simulink model "rosplotlive2018a"  (R2018a)
settings: Solver=VariableStepAuto  StartTime=0.0  StopTime=inf  RelTol=1e-3
undefined symbols (not defined in the file or in its folder): KDalt, KDphi, KDtheta, KIalt, KIp, KIphi, KIq, KIr, KItheta, KNalt, KPalt, KPp, KPphi, KPq, KPr, KPtheta
libraries: robotlib x8, aerolibanimutils x1
settings Model: Creator=Luca  LastModifiedBy=Arne
settings DebuggingCC: LibraryContextMissingDiagnostic=warning
settings CodeAppCC: StateflowObjectComments=on

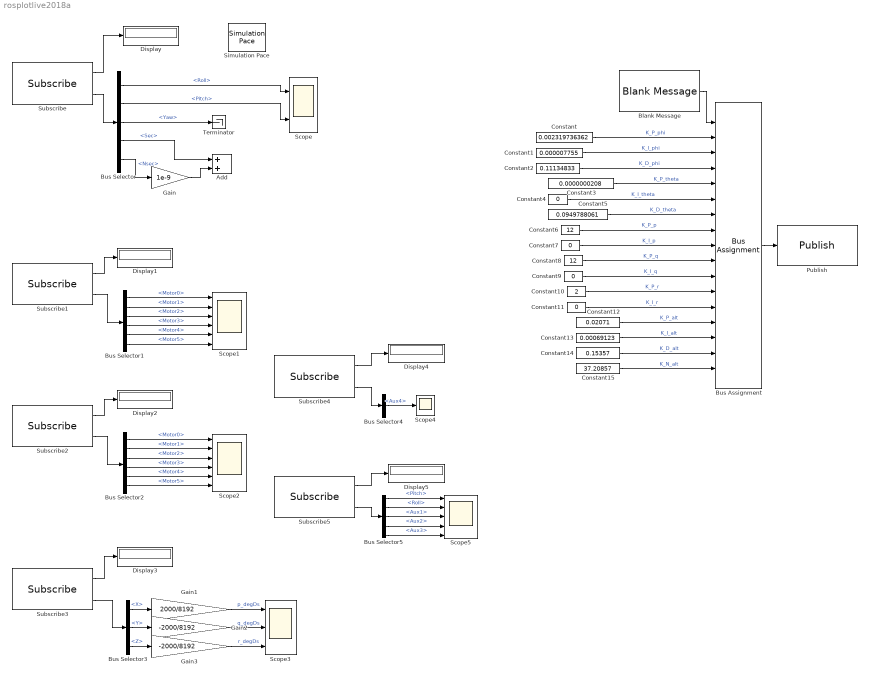
== system rosplotlive2018a ==
  Add : Sum
  Blank Message : robotlib/Blank Message  messageClass=Message  entityType=phx_trajectory_planner/Gains  messageType=phx_trajectory_planner/Gains  SampleTime=inf
      settings: SourceProductBaseCode=RO
  Bus Assignment : BusAssignment  AssignedSignals=KPphi,KIphi,KDphi,KPtheta,KItheta,KDtheta,KPp,KIp,KPq,KIq,KPr,KIr,KPalt,KIalt,KDalt,KNalt
  Bus Selector : BusSelector  OutputSignals=Roll,Pitch,Yaw,Header.Stamp.Sec,Header.Stamp.Nsec
  Bus Selector1 : BusSelector  OutputSignals=Motor0,Motor1,Motor2,Motor3,Motor4,Motor5
  Bus Selector2 : BusSelector  OutputSignals=Motor0,Motor1,Motor2,Motor3,Motor4,Motor5
  Bus Selector3 : BusSelector  OutputSignals=AngularVelocity.X,AngularVelocity.Y,AngularVelocity.Z
  Bus Selector4 : BusSelector  OutputSignals=Aux4
  Bus Selector5 : BusSelector  OutputSignals=Pitch,Roll,Aux1,Aux2,Aux3
  Constant : Constant  Value=0.002319736362
  Constant1 : Constant  Value=0.000007755
  Constant10 : Constant  Value=2
  Constant{4,7,9,11} (4 alike) : Constant  Value=0
  Constant12 : Constant  Value=0.02071
  Constant13 : Constant  Value=0.00069123
  Constant14 : Constant  Value=0.15357
  Constant15 : Constant  Value=37.20857
  Constant2 : Constant  Value=0.11134833
  Constant3 : Constant  Value=0.0000000208
  Constant5 : Constant  Value=0.0949788061
  Constant6 : Constant  Value=12
  Constant8 : Constant  Value=12
  Display{,1..5} (6 alike) : Display
  Gain : Gain  Gain=1e-9
  Gain1 : Gain  Gain=2000/8192
  Gain2 : Gain  Gain=-2000/8192
  Gain3 : Gain  Gain=-2000/8192
  Publish : robotlib/Publish  topicSource=Select from ROS network  topic=/my_topic  messageType=geometry_msgs/Point  messageQueueLength=1
      settings: SourceProductBaseCode=RO
  Scope : Scope  NumInputPorts=2
  Scope1 : Scope  NumInputPorts=6
  Scope2 : Scope  NumInputPorts=6
  Scope3 : Scope  NumInputPorts=3
  Scope4 : Scope
  Scope5 : Scope  NumInputPorts=5
  Simulation Pace : aerolibanimutils/Simulation Pace  SimulationPace=1  SleepMode=MATLAB Thread  OutputPaceError=off  SampleTime=1/30
  Subscribe : robotlib/Subscribe  topicSource=Specify your own  topic=/phx/fc/attitude  messageType=phx_uart_msp_bridge/Attitude  sampleTime=-1  messageQueueLength=1
      settings: SourceProductBaseCode=RO
  Subscribe1 : robotlib/Subscribe  topicSource=Specify your own  topic=/phx/fc/motor_set  messageType=phx_uart_msp_bridge/Motor  sampleTime=-1  messageQueueLength=1
      settings: SourceProductBaseCode=RO
  Subscribe2 : robotlib/Subscribe  topicSource=Specify your own  topic=phx/fc/motor  messageType=phx_uart_msp_bridge/Motor  sampleTime=-1  messageQueueLength=1
      settings: SourceProductBaseCode=RO
  Subscribe3 : robotlib/Subscribe  topicSource=Specify your own  topic=phx/imu  messageType=sensor_msgs/Imu  sampleTime=-1  messageQueueLength=1
      settings: SourceProductBaseCode=RO
  Subscribe4 : robotlib/Subscribe  topicSource=Specify your own  topic=/phx/fc/rc  messageType=phx_uart_msp_bridge/RemoteControl  sampleTime=-1  messageQueueLength=1
      settings: SourceProductBaseCode=RO
  Subscribe5 : robotlib/Subscribe  topicSource=Specify your own  topic=/phx/ssh_rc  messageType=phx_uart_msp_bridge/RemoteControl  sampleTime=-1  messageQueueLength=1
      settings: SourceProductBaseCode=RO
  Terminator : Terminator
  wires:
  Subscribe/2 -> Bus Selector/1
  Subscribe/1 -> Display/1
  Bus Selector/1 -> Scope/1  "<Roll>"
  Bus Selector/2 -> Scope/2  "<Pitch>"
  Bus Selector/3 -> Terminator/1  "<Yaw>"
  Bus Selector/4 -> Add/1  "<Sec>"
  Bus Selector/5 -> Gain/1  "<Nsec>"
  Gain/1 -> Add/2
  Subscribe1/1 -> Display1/1
  Subscribe1/2 -> Bus Selector1/1
  Bus Selector1/1 -> Scope1/1  "<Motor0>"
  Bus Selector1/2 -> Scope1/2  "<Motor1>"
  Bus Selector1/3 -> Scope1/3  "<Motor2>"
  Bus Selector1/4 -> Scope1/4  "<Motor3>"
  Bus Selector1/5 -> Scope1/5  "<Motor4>"
  Bus Selector1/6 -> Scope1/6  "<Motor5>"
  Subscribe2/1 -> Display2/1
  Bus Selector2/1 -> Scope2/1  "<Motor0>"
  Bus Selector2/3 -> Scope2/3  "<Motor2>"
  Bus Selector2/4 -> Scope2/4  "<Motor3>"
  Subscribe2/2 -> Bus Selector2/1
  Bus Selector2/6 -> Scope2/6  "<Motor5>"
  Bus Selector2/2 -> Scope2/2  "<Motor1>"
  Bus Selector2/5 -> Scope2/5  "<Motor4>"
  Subscribe3/1 -> Display3/1
  Subscribe3/2 -> Bus Selector3/1
  Bus Selector3/1 -> Gain1/1  "<X>"
  Bus Selector3/2 -> Gain2/1  "<Y>"
  Bus Selector3/3 -> Gain3/1  "<Z>"
  Gain1/1 -> Scope3/1  "p_degDs"
  Gain2/1 -> Scope3/2  "q_degDs"
  Gain3/1 -> Scope3/3  "r_degDs"
  Subscribe4/1 -> Display4/1
  Subscribe4/2 -> Bus Selector4/1
  Bus Selector4/1 -> Scope4/1  "<Aux4>"
  Subscribe5/1 -> Display5/1
  Subscribe5/2 -> Bus Selector5/1
  Bus Selector5/1 -> Scope5/1  "<Pitch>"
  Bus Selector5/2 -> Scope5/2  "<Roll>"
  Bus Selector5/3 -> Scope5/3  "<Aux1>"
  Bus Selector5/4 -> Scope5/4  "<Aux2>"
  Bus Selector5/5 -> Scope5/5  "<Aux3>"
  Constant/1 -> Bus Assignment/2  "K_P_phi"
  Constant1/1 -> Bus Assignment/3  "K_I_phi"
  Constant2/1 -> Bus Assignment/4  "K_D_phi"
  Constant3/1 -> Bus Assignment/5  "K_P_theta"
  Constant4/1 -> Bus Assignment/6  "K_I_theta"
  Constant5/1 -> Bus Assignment/7  "K_D_theta"
  Constant6/1 -> Bus Assignment/8  "K_P_p"
  Constant7/1 -> Bus Assignment/9  "K_I_p"
  Constant8/1 -> Bus Assignment/10  "K_P_q"
  Constant9/1 -> Bus Assignment/11  "K_I_q"
  Constant10/1 -> Bus Assignment/12  "K_P_r"
  Constant11/1 -> Bus Assignment/13  "K_I_r"
  Constant13/1 -> Bus Assignment/15  "K_I_alt"
  Constant14/1 -> Bus Assignment/16  "K_D_alt"
  Constant12/1 -> Bus Assignment/14  "K_P_alt"
  Constant15/1 -> Bus Assignment/17  "K_N_alt"
  Bus Assignment/1 -> Publish/1
  Blank Message/1 -> Bus Assignment/1
